simulink model "DYNctl_ver4_etud_obfusc"  (R2020b)
settings: Solver=ode45  StartTime=0.0  StopTime=tfin  FixedStep=0.001  RelTol=1e-09  EnableMultiTasking=on
undefined symbols (not defined in the file or in its folder): A_Ax, A_Ay, A_Az, A_Px, A_Py, B_Ax, B_Ay, B_Az, B_Px, B_Py, C_Ax, C_Ay, C_Az, C_Px, C_Py, D_Ax, D_Ay, D_Az, D_Px, D_Py, Px_e, Py_e, Va_e, Vb_e, Vc_e, Vx_e, Vy_e, XA, XB, XC, XD, XE, XF, YB, YC, YD, YE, YF, zD_e, zE_e, zF_e
settings Model: Creator=delafontaine  LastModifiedBy=Alexi
settings SolverCC: AlgebraicLoopSolver=LineSearch
settings DataIOCC: LimitDataPoints=on  SaveFormat=Array  SignalLoggingSaveFormat=ModelDataLogs  ReturnWorkspaceOutputs=off
settings OptimizationCC: LifeSpan=inf
settings DebuggingCC: UnderspecifiedInitializationDetection=Classic  MergeDetectMultiDrivingBlocksExec=none  MultiTaskDSMMsg=warning  MultiTaskCondExecSysMsg=none  SFUnexpectedBacktrackingDiag=warning  SFNoUnconditionalDefaultTransitionDiag=warning  SFExecutionAtInitializationDiag=none  ArithmeticOperatorsInVariantConditions=warning
settings HardwareCC: ProdBitPerPointer=32  ProdBitPerSizeT=32  ProdBitPerPtrDiffT=32  ProdLargestAtomicFloat=None  ProdIntDivRoundTo=Undefined  ProdEndianess=Unspecified  ProdWordSize=32  ProdHWDeviceType=32-bit Generic
settings ModelReferenceCC: PropagateSignalLabelsOutOfModel=off
settings SFSimCC: SimUseLocalCustomCode=off  CustomCodeUndefinedFunction=UseInterfaceOnly
settings RTWCC: RTWUseLocalCustomCode=off
settings CodeAppCC: StateflowObjectComments=on
settings GRTTargetCC: TargetLangStandard=C89/C90 (ANSI)
settings ConfigComp: CovMetricSettings=dw  CovSaveCumulativeToWorkspaceVar=on  CovSaveSingleToWorkspaceVar=on  CovExternalEMLEnable=off  CovSFcnEnable=off

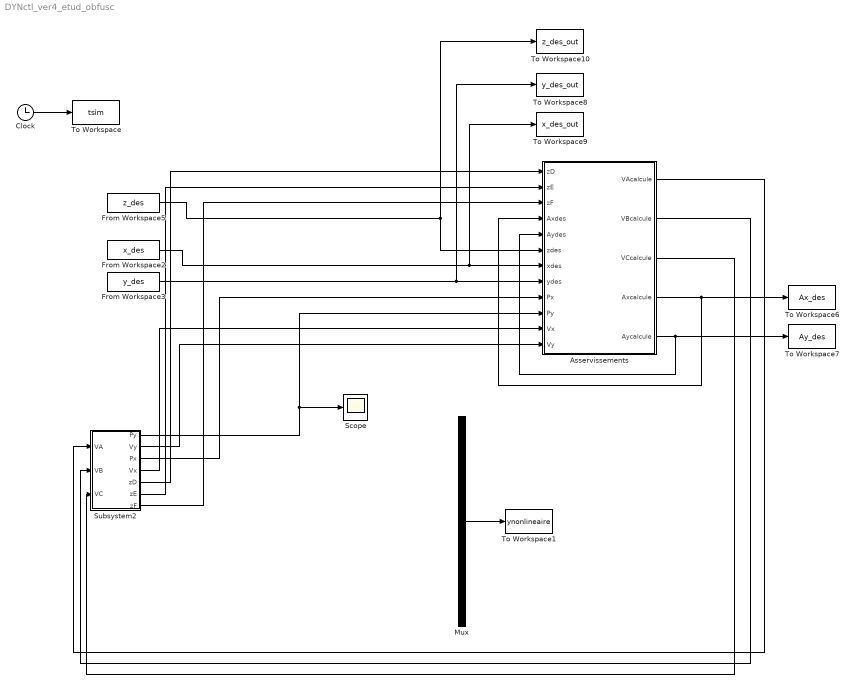
== system DYNctl_ver4_etud_obfusc ==
  Asservissements : Subsystem
      mask help: Simulink:masks:GenSFuncDesc_MD
      mask Help: eval('feval(''rtwprivate'',''rtwhelpview'',''rtw_sfcn_block'')');
  Clock : Clock
  From Workspace2 : FromWorkspace  VariableName=x_des  Interpolate=off  OutputAfterFinalValue=Holding final value
  From Workspace3 : FromWorkspace  VariableName=y_des  Interpolate=off  OutputAfterFinalValue=Holding final value
  From Workspace5 : FromWorkspace  VariableName=z_des  Interpolate=off  OutputAfterFinalValue=Holding final value
  Mux : Mux  Inputs=25
  Scope : Scope
  Subsystem2 : Subsystem
  To Workspace : ToWorkspace  VariableName=tsim  SampleTime=-1
  To Workspace1 : ToWorkspace  VariableName=ynonlineaire  SampleTime=-1
  To Workspace10 : ToWorkspace  VariableName=z_des_out  SampleTime=-1
  To Workspace6 : ToWorkspace  VariableName=Ax_des  SampleTime=-1
  To Workspace7 : ToWorkspace  VariableName=Ay_des  SampleTime=-1
  To Workspace8 : ToWorkspace  VariableName=y_des_out  SampleTime=-1
  To Workspace9 : ToWorkspace  VariableName=x_des_out  SampleTime=-1
  wires:
  Mux/1 -> To Workspace1/1
  Clock/1 -> To Workspace/1
  From Workspace5/1 -> Asservissements/6(zdes), To Workspace10/1
  From Workspace3/1 -> Asservissements/8(ydes), To Workspace8/1
  From Workspace2/1 -> Asservissements/7(xdes), To Workspace9/1
  Asservissements/4(Axcalcule) -> Asservissements/4(Axdes), To Workspace6/1
  Asservissements/5(Aycalcule) -> Asservissements/5(Aydes), To Workspace7/1
  Asservissements/1(VAcalcule) -> Subsystem2/1(VA)
  Asservissements/2(VBcalcule) -> Subsystem2/2(VB)
  Asservissements/3(VCcalcule) -> Subsystem2/3(VC)
  Subsystem2/1(Py) -> Scope/1, Asservissements/10(Py)
  Subsystem2/3(Px) -> Asservissements/9(Px)
  Subsystem2/2(Vy) -> Asservissements/12(Vy)
  Subsystem2/4(Vx) -> Asservissements/11(Vx)
  Subsystem2/5(zD) -> Asservissements/1(zD)
  Subsystem2/6(zE) -> Asservissements/2(zE)
  Subsystem2/7(zF) -> Asservissements/3(zF)

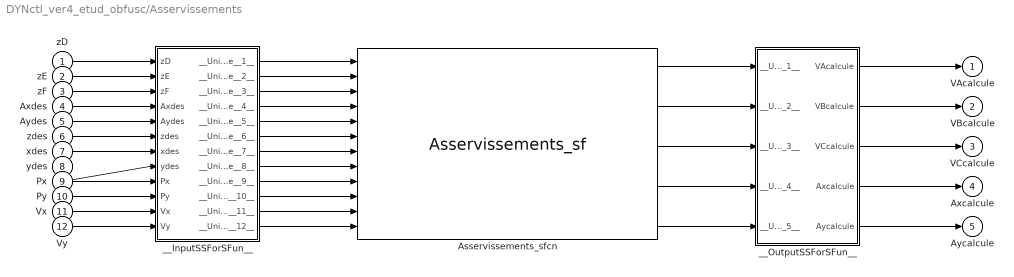
== system DYNctl_ver4_etud_obfusc/Asservissements ==
  zD : Inport
  zE : Inport  Port=2
  zF : Inport  Port=3
  Axdes : Inport  Port=4
  Aydes : Inport  Port=5
  zdes : Inport  Port=6
  xdes : Inport  Port=7
  ydes : Inport  Port=8
  Px : Inport  Port=9
  Py : Inport  Port=10
  Vx : Inport  Port=11
  Vy : Inport  Port=12
  Asservissements_sfcn : S-Function  FunctionName=Asservissements_sf  SFunctionModules=""  SFunctionDeploymentMode=off  EnableBusSupport=off  mask{rtw_sf_name=Asservissements_sf, showVar=off}
      mask prompts: rtw_sf_name "Simulink:masks:GenSFuncName_MP"; showVar "Simulink:masks:GenSFuncShowModuleList_MP"
      mask help: Simulink:masks:GenSFuncDesc_MD
      mask init:
      | displist = '';
      | if ~strcmp(get_param(gcb, 'FunctionName'), rtw_sf_name);
      |   set_param(gcb, 'FunctionName', rtw_sf_name);
      | end
      | % Check if we are generating code
      | rtw_mode = false;
      | if strcmpi(get_param(bdroot(gcb),'SimulationStatus'),'Initializing')
      | 	rtw_mode = strcmpi(get_param(bdroot(gcb),'BuildingRTWCode'),'on') && ...
      | 		~strcmpi(get_param(bdroot(gcb),'TargetStyle'),'SimulationTarget');
      | end
      | if showVar || rtw_mode
      | 	if exist('rtwsfunc') == 2 | exist('rtwsfunc') == 6
      | 		tmplist = rtwsfunc(rtw_sf_name,gcb);
      | 		tmplist = DAStudio.message('Simulink:masks:GenSFuncListOfModules_IC', tmplist);
      | 	elseif showVar
      | 		tmplist1 = DAStudio.message('Simulink:masks:GenSFuncListOfModules_IC', '');
      |         tmplist2 = DAStudio.message('Simulink:masks:GenSFuncNotLicensed_IC');
      |         tmplist = [tmplist1 tmplist2];
      |  	end
      | end
      | if showVar
      |   displist = tmplist;
      | end
      settings: CopyFcn=|
      | if ~strcmp(get_param(gcb,'Linkstatus'),'none') && ...
      | ~strcmp(get_param(gcb,'Linkstatus'),'implicit')
      |   set_param(gcb,'LinkStatus','none');
      | end
      mask Help: eval('feval(''rtwprivate'',''rtwhelpview'',''rtw_sfcn_block'')');
      mask Display:
      | port_label('input',1,'zD');
      | port_label('input',2,'zE');
      | port_label('input',3,'zF');
      | port_label('input',4,'Axdes');
      | port_label('input',5,'Aydes');
      | port_label('input',6,'zdes');
      | port_label('input',7,'xdes');
      | port_label('input',8,'ydes');
      | port_label('input',9,'Px');
      | port_label('input',10,'Py');
      | port_label('input',11,'Vx');
      | port_label('input',12,'Vy');
      | port_label('output',1,'VAcalcule');
      | port_label('output',2,'VBcalcule');
      | port_label('output',3,'VCcalcule');
      | port_label('output',4,'Axcalcule');
      | port_label('output',5,'Aycalcule');
  __InputSSForSFun__ : Subsystem
  __OutputSSForSFun__ : Subsystem
  VAcalcule : Outport
  VBcalcule : Outport  Port=2
  VCcalcule : Outport  Port=3
  Axcalcule : Outport  Port=4
  Aycalcule : Outport  Port=5
  wires:
  zD/1 -> __InputSSForSFun__/1(zD)
  zE/1 -> __InputSSForSFun__/2(zE)
  zF/1 -> __InputSSForSFun__/3(zF)
  Axdes/1 -> __InputSSForSFun__/4(Axdes)
  Aydes/1 -> __InputSSForSFun__/5(Aydes)
  zdes/1 -> __InputSSForSFun__/6(zdes)
  xdes/1 -> __InputSSForSFun__/7(xdes)
  ydes/1 -> __InputSSForSFun__/8(ydes)
  Px/1 -> __InputSSForSFun__/9(Px)
  Py/1 -> __InputSSForSFun__/10(Py)
  Vx/1 -> __InputSSForSFun__/11(Vx)
  Vy/1 -> __InputSSForSFun__/12(Vy)
  __InputSSForSFun__/1(__UniqueOutportName__1__) -> Asservissements_sfcn/1
  __InputSSForSFun__/2(__UniqueOutportName__2__) -> Asservissements_sfcn/2
  __InputSSForSFun__/3(__UniqueOutportName__3__) -> Asservissements_sfcn/3
  __InputSSForSFun__/4(__UniqueOutportName__4__) -> Asservissements_sfcn/4
  __InputSSForSFun__/5(__UniqueOutportName__5__) -> Asservissements_sfcn/5
  __InputSSForSFun__/6(__UniqueOutportName__6__) -> Asservissements_sfcn/6
  __InputSSForSFun__/7(__UniqueOutportName__7__) -> Asservissements_sfcn/7
  __InputSSForSFun__/8(__UniqueOutportName__8__) -> Asservissements_sfcn/8
  __InputSSForSFun__/9(__UniqueOutportName__9__) -> Asservissements_sfcn/9
  __InputSSForSFun__/10(__UniqueOutportName__10__) -> Asservissements_sfcn/10
  __InputSSForSFun__/11(__UniqueOutportName__11__) -> Asservissements_sfcn/11
  __InputSSForSFun__/12(__UniqueOutportName__12__) -> Asservissements_sfcn/12
  Asservissements_sfcn/1 -> __OutputSSForSFun__/1(__UniqueInportName__1__)
  Asservissements_sfcn/2 -> __OutputSSForSFun__/2(__UniqueInportName__2__)
  Asservissements_sfcn/3 -> __OutputSSForSFun__/3(__UniqueInportName__3__)
  Asservissements_sfcn/4 -> __OutputSSForSFun__/4(__UniqueInportName__4__)
  Asservissements_sfcn/5 -> __OutputSSForSFun__/5(__UniqueInportName__5__)
  __OutputSSForSFun__/1(VAcalcule) -> VAcalcule/1
  __OutputSSForSFun__/2(VBcalcule) -> VBcalcule/1
  __OutputSSForSFun__/3(VCcalcule) -> VCcalcule/1
  __OutputSSForSFun__/4(Axcalcule) -> Axcalcule/1
  __OutputSSForSFun__/5(Aycalcule) -> Aycalcule/1

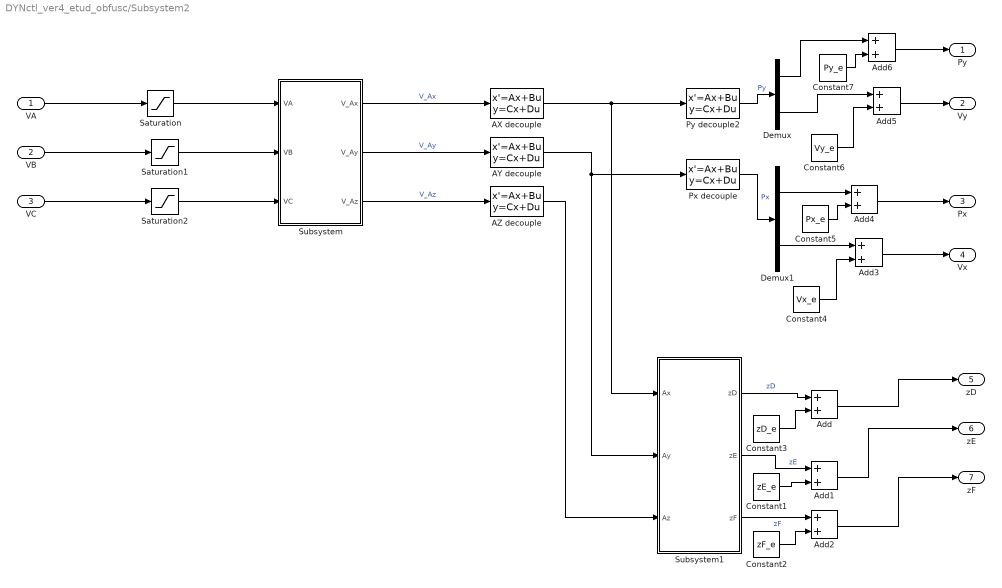
== system DYNctl_ver4_etud_obfusc/Subsystem2 ==
  VA : Inport
  VB : Inport  Port=2
  VC : Inport  Port=3
  AX decouple : StateSpace  A=A_Ax  B=B_Ax  C=C_Ax  D=D_Ax  InitialCondition=0
  AY decouple : StateSpace  A=A_Ay  B=B_Ay  C=C_Ay  D=D_Ay  InitialCondition=0
  AZ decouple : StateSpace  A=A_Az  B=B_Az  C=C_Az  D=D_Az  InitialCondition=0
  Add{,1..6} (7 alike) : Sum
  Constant1 : Constant  Value=zE_e
  Constant2 : Constant  Value=zF_e
  Constant3 : Constant  Value=zD_e
  Constant4 : Constant  Value=Vx_e
  Constant5 : Constant  Value=Px_e
  Constant6 : Constant  Value=Vy_e
  Constant7 : Constant  Value=Py_e
  Demux : Demux  Outputs=2
  Demux1 : Demux  Outputs=2
  Px decouple : StateSpace  A=A_Px  B=B_Px  C=C_Px  D=D_Px  InitialCondition=0
  Py decouple2 : StateSpace  A=A_Py  B=B_Py  C=C_Py  D=D_Py  InitialCondition=0
  Saturation : Saturate  UpperLimit=22  LowerLimit=-22
  Saturation1 : Saturate  UpperLimit=22  LowerLimit=-22
  Saturation2 : Saturate  UpperLimit=22  LowerLimit=-22
  Subsystem : Subsystem
  Subsystem1 : Subsystem
  Py : Outport
  Vy : Outport  Port=2
  Px : Outport  Port=3
  Vx : Outport  Port=4
  zD : Outport  Port=5
  zE : Outport  Port=6
  zF : Outport  Port=7
  wires:
  Subsystem/2(V_Ay) -> AY decouple/1  "V_Ay"
  AX decouple/1 -> Subsystem1/1(Ax), Py decouple2/1
  Subsystem/3(V_Az) -> AZ decouple/1  "V_Az"
  Subsystem/1(V_Ax) -> AX decouple/1  "V_Ax"
  AZ decouple/1 -> Subsystem1/3(Az)
  AY decouple/1 -> Subsystem1/2(Ay), Px decouple/1
  VA/1 -> Saturation/1
  VB/1 -> Saturation1/1
  VC/1 -> Saturation2/1
  Py decouple2/1 -> Demux/1  "Py"
  Px decouple/1 -> Demux1/1  "Px"
  Subsystem1/1(zD) -> Add/1  "zD"
  Constant3/1 -> Add/2
  Constant1/1 -> Add1/2
  Subsystem1/2(zE) -> Add1/1  "zE"
  Subsystem1/3(zF) -> Add2/1  "zF"
  Constant2/1 -> Add2/2
  Add2/1 -> zF/1
  Add1/1 -> zE/1
  Add/1 -> zD/1
  Constant4/1 -> Add3/2
  Demux1/2 -> Add3/1
  Demux1/1 -> Add4/1
  Constant5/1 -> Add4/2
  Constant7/1 -> Add6/2
  Constant6/1 -> Add5/2
  Demux/1 -> Add6/1
  Demux/2 -> Add5/1
  Add6/1 -> Py/1
  Add5/1 -> Vy/1
  Add3/1 -> Vx/1
  Add4/1 -> Px/1
  Saturation/1 -> Subsystem/1(VA)
  Saturation1/1 -> Subsystem/2(VB)
  Saturation2/1 -> Subsystem/3(VC)

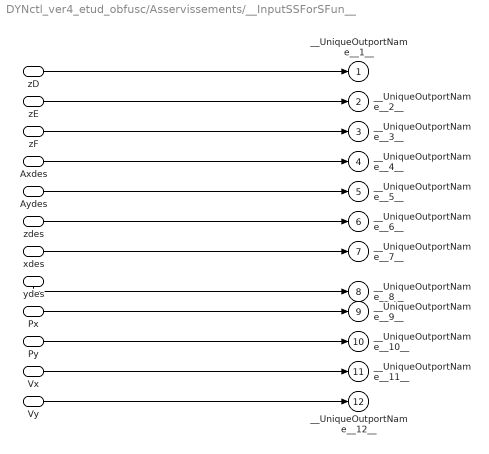
== system DYNctl_ver4_etud_obfusc/Asservissements/__InputSSForSFun__ ==
  zD : Inport
  zE : Inport  Port=2
  zF : Inport  Port=3
  Axdes : Inport  Port=4
  Aydes : Inport  Port=5
  zdes : Inport  Port=6
  xdes : Inport  Port=7
  ydes : Inport  Port=8
  Px : Inport  Port=9
  Py : Inport  Port=10
  Vx : Inport  Port=11
  Vy : Inport  Port=12
  __UniqueOutportName__1__ : Outport
  __UniqueOutportName__2__ : Outport  Port=2
  __UniqueOutportName__3__ : Outport  Port=3
  __UniqueOutportName__4__ : Outport  Port=4
  __UniqueOutportName__5__ : Outport  Port=5
  __UniqueOutportName__6__ : Outport  Port=6
  __UniqueOutportName__7__ : Outport  Port=7
  __UniqueOutportName__8__ : Outport  Port=8
  __UniqueOutportName__9__ : Outport  Port=9
  __UniqueOutportName__10__ : Outport  Port=10
  __UniqueOutportName__11__ : Outport  Port=11
  __UniqueOutportName__12__ : Outport  Port=12
  wires:
  zD/1 -> __UniqueOutportName__1__/1
  zE/1 -> __UniqueOutportName__2__/1
  zF/1 -> __UniqueOutportName__3__/1
  Axdes/1 -> __UniqueOutportName__4__/1
  Aydes/1 -> __UniqueOutportName__5__/1
  zdes/1 -> __UniqueOutportName__6__/1
  xdes/1 -> __UniqueOutportName__7__/1
  ydes/1 -> __UniqueOutportName__8__/1
  Px/1 -> __UniqueOutportName__9__/1
  Py/1 -> __UniqueOutportName__10__/1
  Vx/1 -> __UniqueOutportName__11__/1
  Vy/1 -> __UniqueOutportName__12__/1

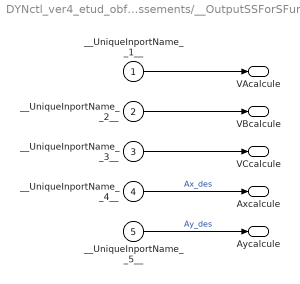
== system DYNctl_ver4_etud_obfusc/Asservissements/__OutputSSForSFun__ ==
  __UniqueInportName__1__ : Inport
  __UniqueInportName__2__ : Inport  Port=2
  __UniqueInportName__3__ : Inport  Port=3
  __UniqueInportName__4__ : Inport  Port=4
  __UniqueInportName__5__ : Inport  Port=5
  VAcalcule : Outport
  VBcalcule : Outport  Port=2
  VCcalcule : Outport  Port=3
  Axcalcule : Outport  Port=4
  Aycalcule : Outport  Port=5
  wires:
  __UniqueInportName__1__/1 -> VAcalcule/1
  __UniqueInportName__2__/1 -> VBcalcule/1
  __UniqueInportName__3__/1 -> VCcalcule/1
  __UniqueInportName__4__/1 -> Axcalcule/1  "Ax_des"
  __UniqueInportName__5__/1 -> Aycalcule/1  "Ay_des"

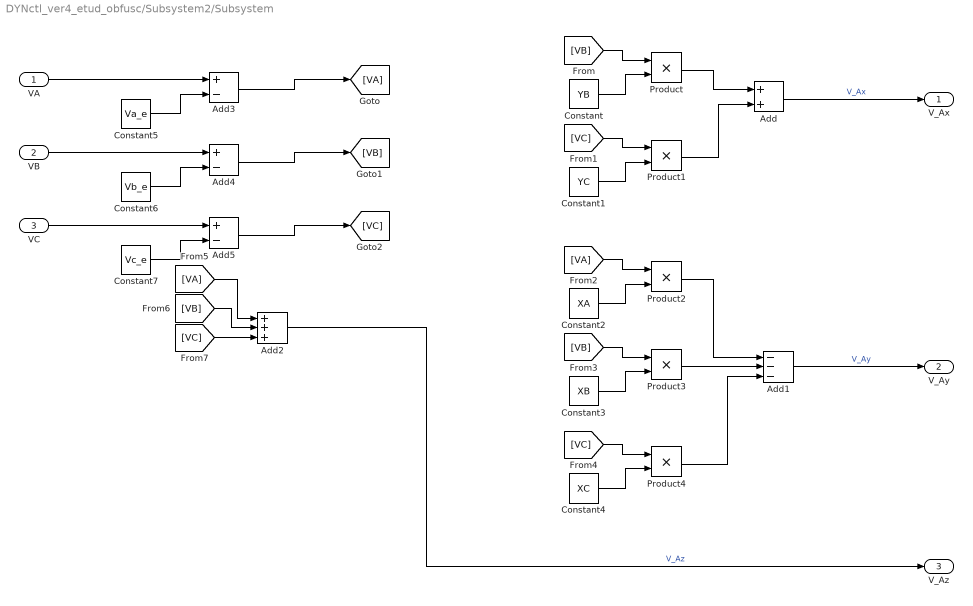
== system DYNctl_ver4_etud_obfusc/Subsystem2/Subsystem ==
  VA : Inport
  VB : Inport  Port=2
  VC : Inport  Port=3
  Add : Sum
  Add1 : Sum  Inputs=---
  Add2 : Sum  Inputs=+++
  Add3 : Sum  Inputs=+-
  Add4 : Sum  Inputs=+-
  Add5 : Sum  Inputs=+-
  Constant : Constant  Value=YB
  Constant1 : Constant  Value=YC
  Constant2 : Constant  Value=XA
  Constant3 : Constant  Value=XB
  Constant4 : Constant  Value=XC
  Constant5 : Constant  Value=Va_e
  Constant6 : Constant  Value=Vb_e
  Constant7 : Constant  Value=Vc_e
  Product{,1..4} (5 alike) : Product
  V_Ax : Outport
  V_Ay : Outport  Port=2
  V_Az : Outport  Port=3
  wires:
  Add2/1 -> V_Az/1  "V_Az"
  Constant4/1 -> Product4/2
  [VA] -> Add2/1
  [VC] -> Product1/1
  Product4/1 -> Add1/3
  Constant1/1 -> Product1/2
  Product2/1 -> Add1/1
  [VB] -> Product3/1
  [VC] -> Product4/1
  [VC] -> Add2/3
  [VB] -> Add2/2
  Constant2/1 -> Product2/2
  Constant3/1 -> Product3/2
  [VA] -> Product2/1
  Product3/1 -> Add1/2
  Product1/1 -> Add/2
  [VB] -> Product/1
  Product/1 -> Add/1
  Constant/1 -> Product/2
  Add/1 -> V_Ax/1  "V_Ax"
  Add1/1 -> V_Ay/1  "V_Ay"
  VA/1 -> Add3/1
  Add3/1 -> [VA]
  Constant5/1 -> Add3/2
  VB/1 -> Add4/1
  Constant6/1 -> Add4/2
  Add4/1 -> [VB]
  VC/1 -> Add5/1
  Constant7/1 -> Add5/2
  Add5/1 -> [VC]

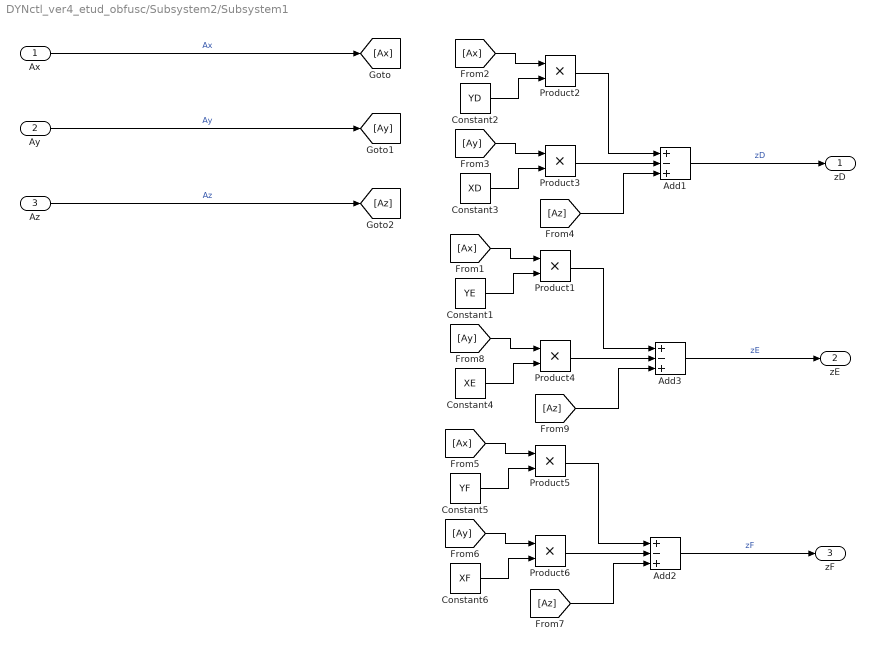
== system DYNctl_ver4_etud_obfusc/Subsystem2/Subsystem1 ==
  Ax : Inport
  Ay : Inport  Port=2
  Az : Inport  Port=3
  Add1 : Sum  Inputs=+-+
  Add2 : Sum  Inputs=+-+
  Add3 : Sum  Inputs=+-+
  Constant1 : Constant  Value=YE
  Constant2 : Constant  Value=YD
  Constant3 : Constant  Value=XD
  Constant4 : Constant  Value=XE
  Constant5 : Constant  Value=YF
  Constant6 : Constant  Value=XF
  Product{1..6} (6 alike) : Product
  zD : Outport
  zE : Outport  Port=2
  zF : Outport  Port=3
  wires:
  [Az] -> Add1/3
  Az/1 -> [Az]  "Az"
  Ax/1 -> [Ax]  "Ax"
  Product2/1 -> Add1/1
  [Ay] -> Product3/1
  Constant2/1 -> Product2/2
  Constant3/1 -> Product3/2
  [Ax] -> Product2/1
  Product3/1 -> Add1/2
  Ay/1 -> [Ay]  "Ay"
  Add1/1 -> zD/1  "zD"
  Product4/1 -> Add3/2
  Constant4/1 -> Product4/2
  [Ax] -> Product1/1
  [Az] -> Add3/3
  [Ay] -> Product4/1
  Add3/1 -> zE/1  "zE"
  Constant1/1 -> Product1/2
  Product1/1 -> Add3/1
  Constant6/1 -> Product6/2
  [Az] -> Add2/3
  [Ay] -> Product6/1
  Product6/1 -> Add2/2
  Product5/1 -> Add2/1
  Constant5/1 -> Product5/2
  Add2/1 -> zF/1  "zF"
  [Ax] -> Product5/1
